simulink model "Mdl_Gear"  (R2024b)
settings: Solver=FixedStepDiscrete  StartTime=0.0  StopTime=10.0  FixedStep=0.1  RelTol=1e-3  EnableMultiTasking=on
values from neighbouring files (symbols this model uses):
  GEAR_MODE_OFF = mpt.Parameter    [Mdl_Gear_DD.m]
  GEAR_STATUS_OFF = mpt.Parameter    [Mdl_Gear_DD.m]
  HMI_READY = mpt.Parameter    [Mdl_Gear_DD.m]
  IND_FLASH_1HZ = mpt.Parameter    [Mdl_Gear_DD.m]
  IND_FLASH_4HZ = mpt.Parameter    [Mdl_Gear_DD.m]
  IND_TURN_OFF = mpt.Parameter    [Mdl_Gear_DD.m]
  Init_Count = mpt.Parameter    [Mdl_Gear_DD.m]
  Mdl_Gear_cTaskPeriod = mpt.Parameter    [Mdl_Gear_rte_types.m]
  PGM_LOGIC_ENABLE = mpt.Parameter    [Mdl_Gear_DD.m]
  RTE_E_MAX_AGE_EXCEEDED = mpt.Parameter    [Mdl_Gear_rte_types.m]
  RTE_E_NEVER_RECEIVED = mpt.Parameter    [Mdl_Gear_rte_types.m]
  Shift_Blink_P1 = mpt.Parameter    [Mdl_Gear_DD.m]
  Shift_Blink_P2 = mpt.Parameter    [Mdl_Gear_DD.m]
  STATUS_OFF = mpt.Parameter    [Mdl_Gear_DD.m]
  STATUS_ON = mpt.Parameter    [Mdl_Gear_DD.m]
  Timer_Param = mpt.Parameter    [Mdl_Gear_DD.m]
  TYPE1 = mpt.Parameter    [Mdl_Gear_DD.m]
  TYPE1_SBW = mpt.Parameter    [Mdl_Gear_DD.m]
  TYPE2 = mpt.Parameter    [Mdl_Gear_DD.m]
  TYPE2_MECH = mpt.Parameter    [Mdl_Gear_DD.m]
  TYPE3 = mpt.Parameter    [Mdl_Gear_DD.m]
  VALUE_FIFTEEN = mpt.Parameter    [Mdl_Gear_DD.m]
  VALUE_FIVE = mpt.Parameter    [Mdl_Gear_DD.m]
  VALUE_FOUR = mpt.Parameter    [Mdl_Gear_DD.m]
  VALUE_ONE = mpt.Parameter    [Mdl_Gear_DD.m]
  VALUE_TEN = mpt.Parameter    [Mdl_Gear_DD.m]
  VALUE_THREE = mpt.Parameter    [Mdl_Gear_DD.m]
  VALUE_TWO = mpt.Parameter    [Mdl_Gear_DD.m]
  VALUE_ZERO = mpt.Parameter    [Mdl_Gear_DD.m]
undefined symbols (not defined in the file or in its folder): CLUSTER_INACTIVE, eGearIn, eGearModeIn, eGearRecommendationIn, eGearStatusIn, eSIGNAL_MISSING, eSIGNAL_NEVER_RECEIVED, IgnOff, IgnOn, NETWORK_NORMAL, NETWORK_STANDALONE, PTSYS_EV, PTSYS_PHV, tRxSignalId_type_instance, tRxSignalStatus_type_instance
libraries: simulink x9
(part 1 of 2)
settings Model: Creator=AELANGO6  LastModifiedBy=AELANGO6
settings DataIOCC: SaveOutput=off
settings OptimizationCC: DefaultParameterBehavior=Inlined  EnhancedBackFolding=on  PassReuseOutputArgsAs=Individual arguments  ZeroExternalMemoryAtStartup=off  ZeroInternalMemoryAtStartup=off  MaxStackSize=750  RemoveLocalVariableInitialization=off  OptimizeBlockOrder=speed  DifferentSizesBufferReuse=on  OptimizationCustomize=off  EfficientTunableParamExpr=on
settings DebuggingCC: ParameterTunabilityLossMsg=error
settings SFSimCC: MATLABDynamicMemAlloc=off
settings RTWCC: Description=AUTOSAR  SystemTargetFile=autosar.tlc  GenCodeOnly=on  TemplateMakefile=ert_default_tmf  PortableWordSizes=on  DataTypeReplacement=CDataTypesFixedWidth
settings CodeAppCC: ForceParamTrailComments=on  IgnoreCustomStorageClasses=off  OperatorAnnotations=on  SimulinkDataObjDesc=on  SFDataObjDesc=on  InsertBlockDesc=on
settings STFCustomTargetCC: TargetLangStandard=C99 (ISO)  MultiwordLength=256  ParMdlRefBuildCompliant=on  CompOptLevelCompliant=on  IncludeMdlTerminateFcn=off  CombineOutputUpdateFcns=on  SuppressErrorStatus=on  ERTCustomFileBanners=on  SupportNonFinite=off  SupportComplex=off  SupportContinuousTime=off  SupportNonInlinedSFcns=off  RemoveResetFunc=on  ParenthesesLevel=Maximum  CastingMode=Standards  MATLABClassNameForMDSCustomization=Simulink.SoftwareTarget.ERTCustomization  AutosarCompliant=on  UseToolchainInfoCompliant=on  LookupTableObjectStructAxisOrder=2,1,3,4,...  LUTObjectStructOrderEvenSpacing=Size,Table,Breakpoints  SystemTargetFile=autosar.tlc
settings ERTTargetCC: TargetLangStandard=C99 (ISO)  ConcurrentExecutionCompliant=off  IncludeMdlTerminateFcn=off  SuppressErrorStatus=on  SupportNonFinite=off  SupportComplex=off  ParenthesesLevel=Maximum  CastingMode=Standards  ModelStepFunctionPrototypeControlCompliant=off  CPPClassGenCompliant=off  AutosarCompliant=on  LookupTableObjectStructAxisOrder=2,1,3,4,...  LUTObjectStructOrderEvenSpacing=Size,Table,Breakpoints  ERTCustomFileTemplate=example_file_process.tlc  ERTFilePackagingFormat=CompactWithDataFile  BooleanTrueId=TRUE  BooleanFalseId=FALSE

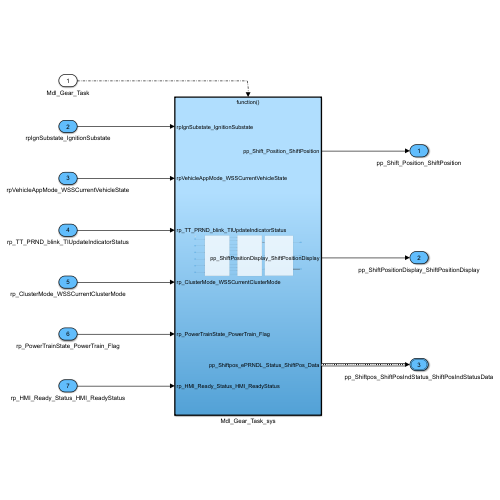
[thumbnail: Simulink's stored preview of the top-level diagram]
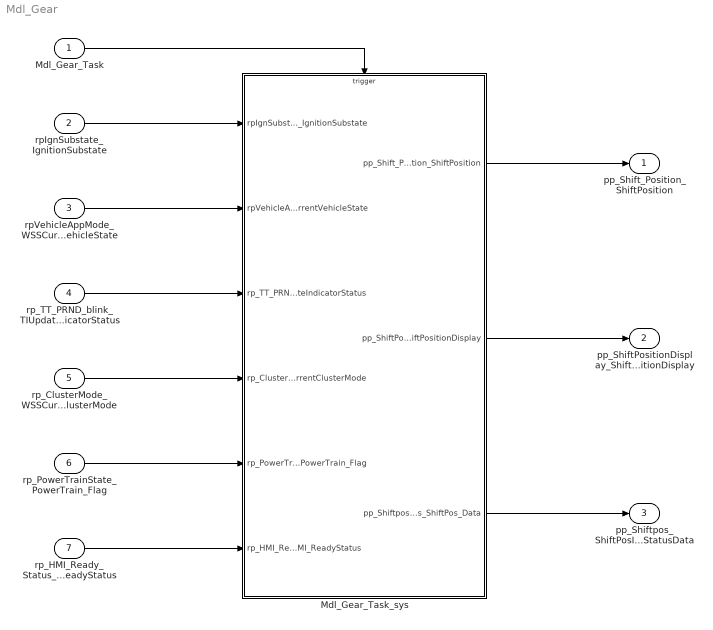
== system Mdl_Gear ==
  Mdl_Gear_Task : Inport  SampleTime=0.1  OutputFunctionCall=on
  rpIgnSubstate_IgnitionSubstate : Inport  Port=2  OutDataTypeStr=IgntionSubstateType  PortDimensions=1
  rpVehicleAppMode_WSSCurrentVehicleState : Inport  Port=3  OutDataTypeStr=VehicleActiveModes  PortDimensions=1
  rp_TT_PRND_blink_TIUpdateIndicatorStatus : Inport  Port=4  OutDataTypeStr=uint8  PortDimensions=1
  rp_ClusterMode_WSSCurrentClusterMode : Inport  Port=5  OutDataTypeStr=ClusterModes  PortDimensions=1
  rp_PowerTrainState_PowerTrain_Flag : Inport  Port=6  OutDataTypeStr=uint8  PortDimensions=1
  rp_HMI_Ready_Status_HMI_ReadyStatus : Inport  Port=7  OutDataTypeStr=HMIReadySts_Type  PortDimensions=1
  Mdl_Gear_Task_sys : Subsystem  TreatAsAtomicUnit=on
  pp_Shift_Position_ShiftPosition : Outport  OutDataTypeStr=ShiftPosition
  pp_ShiftPositionDisplay_ShiftPositionDisplay : Outport  Port=2  OutDataTypeStr=uint8
  pp_Shiftpos_ShiftPosIndStatus_ShiftPosIndStatusData : Outport  Port=3  OutDataTypeStr=Bus:SShiftPosIndStatus
  wires:
  Mdl_Gear_Task/1 -> Mdl_Gear_Task_sys/Trigger
  rp_ClusterMode_WSSCurrentClusterMode/1 -> Mdl_Gear_Task_sys/4(rp_ClusterMode_WSSCurrentClusterMode)
  rpIgnSubstate_IgnitionSubstate/1 -> Mdl_Gear_Task_sys/1(rpIgnSubstate_IgnitionSubstate)
  rpVehicleAppMode_WSSCurrentVehicleState/1 -> Mdl_Gear_Task_sys/2(rpVehicleAppMode_WSSCurrentVehicleState)
  Mdl_Gear_Task_sys/3(pp_Shiftpos_ePRNDL_Status_ShiftPos_Data) -> pp_Shiftpos_ShiftPosIndStatus_ShiftPosIndStatusData/1
  rp_TT_PRND_blink_TIUpdateIndicatorStatus/1 -> Mdl_Gear_Task_sys/3(rp_TT_PRND_blink_TIUpdateIndicatorStatus)
  Mdl_Gear_Task_sys/1(pp_Shift_Position_ShiftPosition) -> pp_Shift_Position_ShiftPosition/1
  rp_PowerTrainState_PowerTrain_Flag/1 -> Mdl_Gear_Task_sys/5(rp_PowerTrainState_PowerTrain_Flag)
  rp_HMI_Ready_Status_HMI_ReadyStatus/1 -> Mdl_Gear_Task_sys/6(rp_HMI_Ready_Status_HMI_ReadyStatus)
  Mdl_Gear_Task_sys/2(pp_ShiftPositionDisplay_ShiftPositionDisplay) -> pp_ShiftPositionDisplay_ShiftPositionDisplay/1

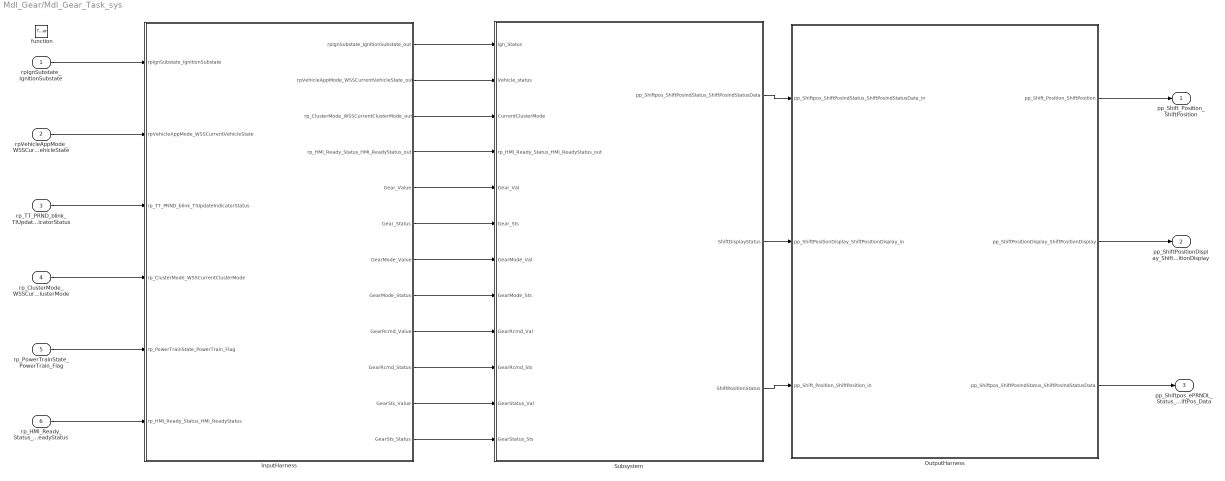
== system Mdl_Gear/Mdl_Gear_Task_sys ==
  rpIgnSubstate_IgnitionSubstate : Inport  OutDataTypeStr=IgntionSubstateType  PortDimensions=1
  rpVehicleAppMode_WSSCurrentVehicleState : Inport  Port=2  OutDataTypeStr=VehicleActiveModes  PortDimensions=1
  rp_TT_PRND_blink_TIUpdateIndicatorStatus : Inport  Port=3  OutDataTypeStr=uint8  PortDimensions=1
  rp_ClusterMode_WSSCurrentClusterMode : Inport  Port=4  OutDataTypeStr=ClusterModes  PortDimensions=1
  rp_PowerTrainState_PowerTrain_Flag : Inport  Port=5  OutDataTypeStr=uint8  PortDimensions=1
  rp_HMI_Ready_Status_HMI_ReadyStatus : Inport  Port=6  OutDataTypeStr=HMIReadySts_Type  PortDimensions=1
  function : TriggerPort  TriggerType=function-call  VariantControl=(inherit)  SampleTimeType=periodic  SampleTime=-1
  InputHarness : Subsystem  Variant=on
  OutputHarness : Subsystem  Variant=on
  Subsystem : Subsystem
  pp_Shift_Position_ShiftPosition : Outport  OutDataTypeStr=ShiftPosition  PortDimensions=1
  pp_ShiftPositionDisplay_ShiftPositionDisplay : Outport  Port=2  OutDataTypeStr=uint8  PortDimensions=1
  pp_Shiftpos_ePRNDL_Status_ShiftPos_Data : Outport  Port=3  OutDataTypeStr=Bus: SShiftPosIndStatus  PortDimensions=1
  wires:
  rpVehicleAppMode_WSSCurrentVehicleState/1 -> InputHarness/2(rpVehicleAppMode_WSSCurrentVehicleState)
  rpIgnSubstate_IgnitionSubstate/1 -> InputHarness/1(rpIgnSubstate_IgnitionSubstate)
  rp_TT_PRND_blink_TIUpdateIndicatorStatus/1 -> InputHarness/3(rp_TT_PRND_blink_TIUpdateIndicatorStatus)
  InputHarness/9(GearRcmd_Value) -> Subsystem/9(GearRcmd_Val)
  rp_ClusterMode_WSSCurrentClusterMode/1 -> InputHarness/4(rp_ClusterMode_WSSCurrentClusterMode)
  InputHarness/8(GearMode_Status) -> Subsystem/8(GearMode_Sts)
  rp_PowerTrainState_PowerTrain_Flag/1 -> InputHarness/5(rp_PowerTrainState_PowerTrain_Flag)
  rp_HMI_Ready_Status_HMI_ReadyStatus/1 -> InputHarness/6(rp_HMI_Ready_Status_HMI_ReadyStatus)
  InputHarness/1(rpIgnSubstate_IgnitionSubstate_out) -> Subsystem/1(Ign_Status)
  InputHarness/2(rpVehicleAppMode_WSSCurrentVehicleState_out) -> Subsystem/2(Vehicle_status)
  InputHarness/10(GearRcmd_Status) -> Subsystem/10(GearRcmd_Sts)
  InputHarness/3(rp_ClusterMode_WSSCurrentClusterMode_out) -> Subsystem/3(CurrentClusterMode)
  InputHarness/4(rp_HMI_Ready_Status_HMI_ReadyStatus_out) -> Subsystem/4(rp_HMI_Ready_Status_HMI_ReadyStatus_out)
  InputHarness/5(Gear_Value) -> Subsystem/5(Gear_Val)
  InputHarness/6(Gear_Status) -> Subsystem/6(Gear_Sts)
  InputHarness/7(GearMode_Value) -> Subsystem/7(GearMode_Val)
  InputHarness/11(GearSts_Value) -> Subsystem/11(GearStatus_Val)
  InputHarness/12(GearSts_Status) -> Subsystem/12(GearStatus_Sts)
  Subsystem/1(pp_Shiftpos_ShiftPosIndStatus_ShiftPosIndStatusData) -> OutputHarness/1(pp_Shiftpos_ShiftPosIndStatus_ShiftPosIndStatusData_in)
  Subsystem/2(ShiftDisplayStatus) -> OutputHarness/2(pp_ShiftPositionDisplay_ShiftPositionDisplay_in)
  Subsystem/3(ShiftPositionStatus) -> OutputHarness/3(pp_Shift_Position_ShiftPosition_in)
  OutputHarness/2(pp_ShiftPositionDisplay_ShiftPositionDisplay) -> pp_ShiftPositionDisplay_ShiftPositionDisplay/1
  OutputHarness/3(pp_Shiftpos_ShiftPosIndStatus_ShiftPosIndStatusData) -> pp_Shiftpos_ePRNDL_Status_ShiftPos_Data/1
  OutputHarness/1(pp_Shift_Position_ShiftPosition) -> pp_Shift_Position_ShiftPosition/1

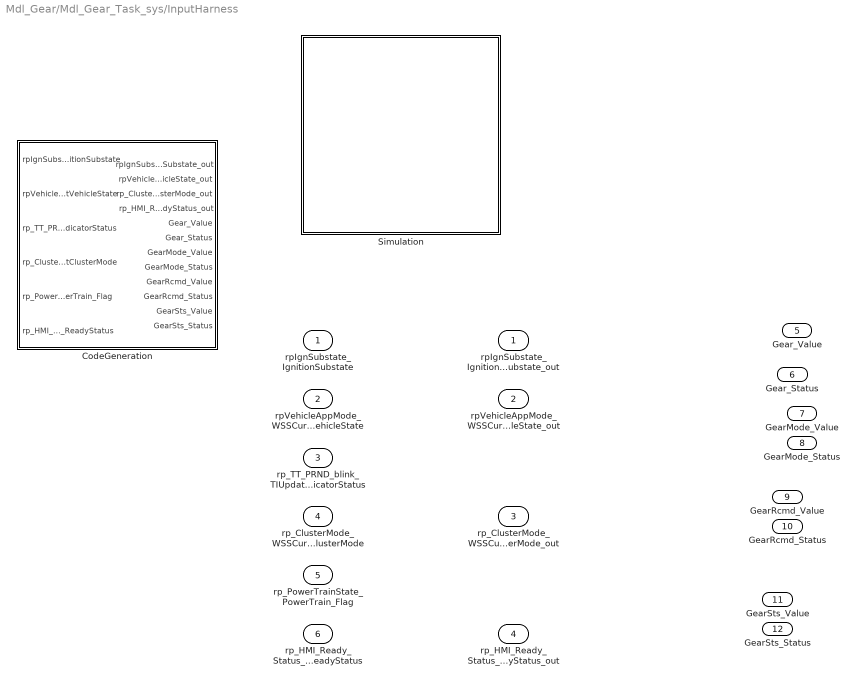
== system Mdl_Gear/Mdl_Gear_Task_sys/InputHarness ==
  rpIgnSubstate_IgnitionSubstate : Inport  OutDataTypeStr=IgntionSubstateType  PortDimensions=1
  rpVehicleAppMode_WSSCurrentVehicleState : Inport  Port=2  OutDataTypeStr=VehicleActiveModes  PortDimensions=1
  rp_TT_PRND_blink_TIUpdateIndicatorStatus : Inport  Port=3  OutDataTypeStr=uint8  PortDimensions=1
  rp_ClusterMode_WSSCurrentClusterMode : Inport  Port=4  OutDataTypeStr=ClusterModes  PortDimensions=1
  rp_PowerTrainState_PowerTrain_Flag : Inport  Port=5  OutDataTypeStr=uint8  PortDimensions=1
  rp_HMI_Ready_Status_HMI_ReadyStatus : Inport  Port=6  OutDataTypeStr=HMIReadySts_Type  PortDimensions=1
  CodeGeneration : Subsystem  VariantControl=CODEGENERATION
  Simulation : Subsystem  VariantControl=SIMULATION
  rpIgnSubstate_IgnitionSubstate_out : Outport  OutDataTypeStr=IgntionSubstateType  PortDimensions=1
  rpVehicleAppMode_WSSCurrentVehicleState_out : Outport  Port=2  OutDataTypeStr=VehicleActiveModes  PortDimensions=1
  rp_ClusterMode_WSSCurrentClusterMode_out : Outport  Port=3  OutDataTypeStr=ClusterModes  PortDimensions=1
  rp_HMI_Ready_Status_HMI_ReadyStatus_out : Outport  Port=4  OutDataTypeStr=HMIReadySts_Type  PortDimensions=1
  Gear_Value : Outport  Port=5
  Gear_Status : Outport  Port=6
  GearMode_Value : Outport  Port=7
  GearMode_Status : Outport  Port=8
  GearRcmd_Value : Outport  Port=9
  GearRcmd_Status : Outport  Port=10
  GearSts_Value : Outport  Port=11
  GearSts_Status : Outport  Port=12

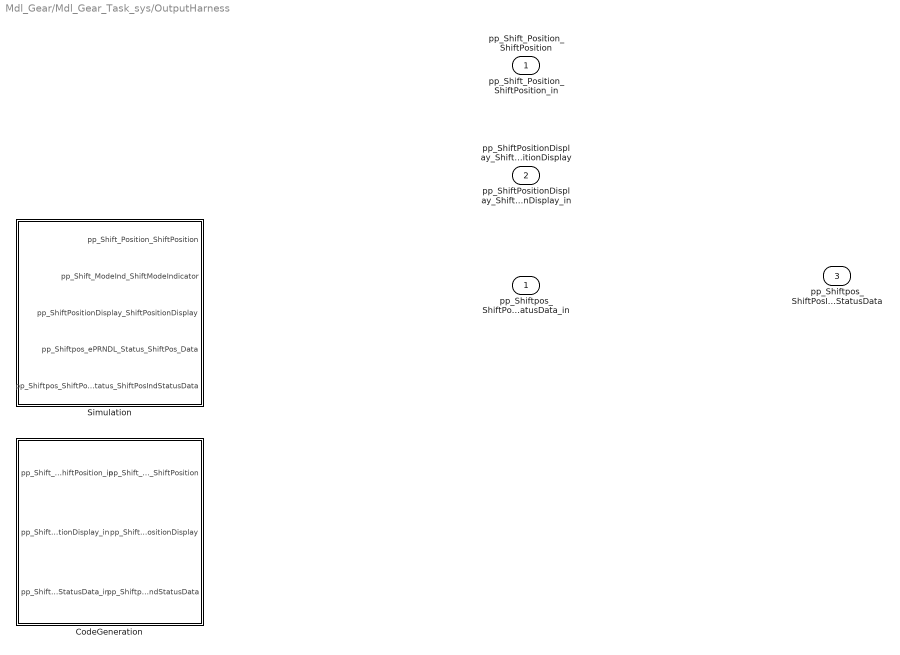
== system Mdl_Gear/Mdl_Gear_Task_sys/OutputHarness ==
  pp_Shiftpos_ShiftPosIndStatus_ShiftPosIndStatusData_in : Inport  OutDataTypeStr=Bus:SShiftPosIndStatus  PortDimensions=1
  pp_ShiftPositionDisplay_ShiftPositionDisplay_in : Inport  Port=2  OutDataTypeStr=uint8  PortDimensions=1
  pp_Shift_Position_ShiftPosition_in : Inport  Port=3  OutDataTypeStr=ShiftPosition  PortDimensions=1
  CodeGeneration : Subsystem  VariantControl=CODEGENERATION
  Simulation : Subsystem  VariantControl=SIMULATION
  pp_Shift_Position_ShiftPosition : Outport  OutDataTypeStr=ShiftPosition  PortDimensions=1
  pp_ShiftPositionDisplay_ShiftPositionDisplay : Outport  Port=2  OutDataTypeStr=uint8  PortDimensions=1
  pp_Shiftpos_ShiftPosIndStatus_ShiftPosIndStatusData : Outport  Port=3  OutDataTypeStr=Bus:SShiftPosIndStatus  PortDimensions=1

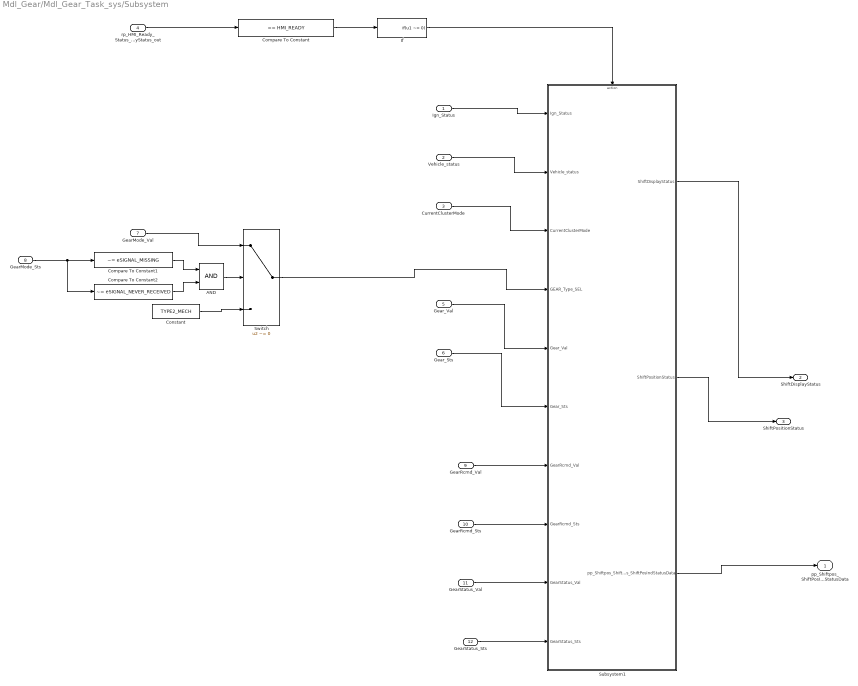
== system Mdl_Gear/Mdl_Gear_Task_sys/Subsystem ==
  Ign_Status : Inport
  Vehicle_status : Inport  Port=2
  CurrentClusterMode : Inport  Port=3
  rp_HMI_Ready_Status_HMI_ReadyStatus_out : Inport  Port=4
  Gear_Val : Inport  Port=5
  Gear_Sts : Inport  Port=6
  GearMode_Val : Inport  Port=7
  GearMode_Sts : Inport  Port=8
  GearRcmd_Val : Inport  Port=9
  GearRcmd_Sts : Inport  Port=10
  GearStatus_Val : Inport  Port=11
  GearStatus_Sts : Inport  Port=12
  AND : Logic  AllPortsSameDT=off  OutDataTypeStr=boolean
  Compare To Constant : simulink/Logic and Bit Operations/Compare To Constant  relop===  const=HMI_READY  OutDataTypeStr=boolean
  Compare To Constant1 : simulink/Logic and Bit Operations/Compare To Constant  relop=~=  const=eSIGNAL_MISSING  OutDataTypeStr=boolean
  Compare To Constant2 : simulink/Logic and Bit Operations/Compare To Constant  relop=~=  const=eSIGNAL_NEVER_RECEIVED  OutDataTypeStr=boolean
  Constant : Constant  Value=TYPE2_MECH
  If : If  IfExpression=u1 ~= 0  ShowElse=off
  Subsystem1 : Subsystem
  Switch : Switch  Criteria=u2 ~= 0  SaturateOnIntegerOverflow=off  InputSameDT=off
  pp_Shiftpos_ShiftPosIndStatus_ShiftPosIndStatusData : Outport  OutDataTypeStr=Bus:SShiftPosIndStatus  PortDimensions=1  VectorParamsAs1DForOutWhenUnconnected=off
  ShiftDisplayStatus : Outport  Port=2  VectorParamsAs1DForOutWhenUnconnected=off
  ShiftPositionStatus : Outport  Port=3  OutDataTypeStr=uint8  VectorParamsAs1DForOutWhenUnconnected=off
  wires:
  Ign_Status/1 -> Subsystem1/1(Ign_Status)
  CurrentClusterMode/1 -> Subsystem1/3(CurrentClusterMode)
  Subsystem1/3(pp_Shiftpos_ShiftPosIndStatus_ShiftPosIndStatusData) -> pp_Shiftpos_ShiftPosIndStatus_ShiftPosIndStatusData/1
  Subsystem1/1(ShiftDisplayStatus) -> ShiftDisplayStatus/1
  Subsystem1/2(ShiftPositionStatus) -> ShiftPositionStatus/1
  rp_HMI_Ready_Status_HMI_ReadyStatus_out/1 -> Compare To Constant/1
  Compare To Constant/1 -> If/1
  If/1 -> Subsystem1/Action
  Vehicle_status/1 -> Subsystem1/2(Vehicle_status)
  Gear_Val/1 -> Subsystem1/5(Gear_Val)
  Gear_Sts/1 -> Subsystem1/6(Gear_Sts)
  GearMode_Val/1 -> Switch/1
  GearMode_Sts/1 -> Compare To Constant2/1, Compare To Constant1/1
  GearRcmd_Val/1 -> Subsystem1/7(GearRcmd_Val)
  GearRcmd_Sts/1 -> Subsystem1/8(GearRcmd_Sts)
  GearStatus_Val/1 -> Subsystem1/9(GearStatus_Val)
  GearStatus_Sts/1 -> Subsystem1/10(GearStatus_Sts)
  Compare To Constant1/1 -> AND/1
  Compare To Constant2/1 -> AND/2
  AND/1 -> Switch/2
  Switch/1 -> Subsystem1/4(GEAR_Type_SEL)
  Constant/1 -> Switch/3

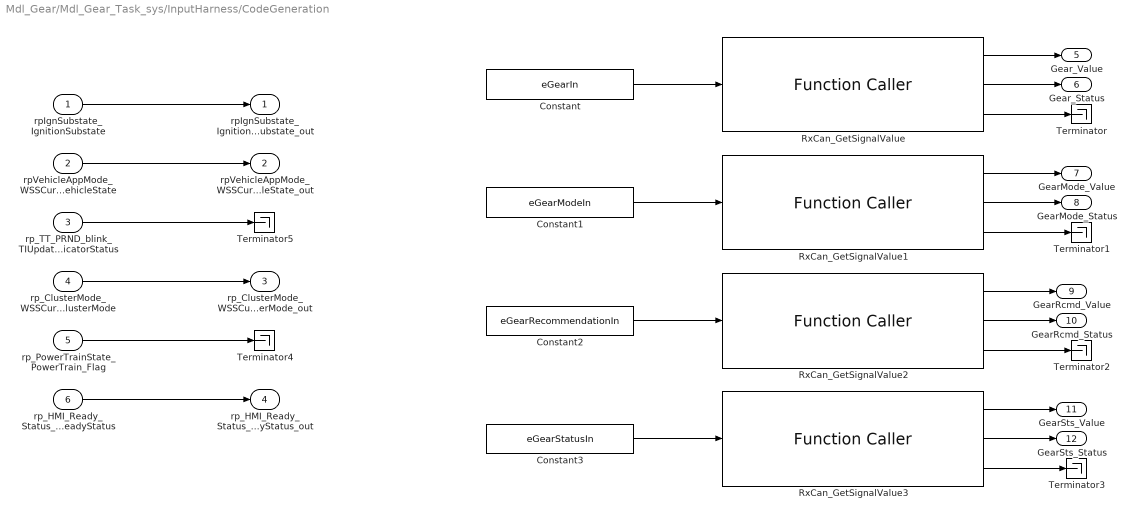
== system Mdl_Gear/Mdl_Gear_Task_sys/InputHarness/CodeGeneration ==
  rpIgnSubstate_IgnitionSubstate : Inport  OutDataTypeStr=IgntionSubstateType  PortDimensions=1
  rpVehicleAppMode_WSSCurrentVehicleState : Inport  Port=2  OutDataTypeStr=VehicleActiveModes  PortDimensions=1
  rp_TT_PRND_blink_TIUpdateIndicatorStatus : Inport  Port=3  OutDataTypeStr=uint8  PortDimensions=1
  rp_ClusterMode_WSSCurrentClusterMode : Inport  Port=4  OutDataTypeStr=ClusterModes  PortDimensions=1
  rp_PowerTrainState_PowerTrain_Flag : Inport  Port=5  OutDataTypeStr=uint8  PortDimensions=1
  rp_HMI_Ready_Status_HMI_ReadyStatus : Inport  Port=6  OutDataTypeStr=HMIReadySts_Type  PortDimensions=1
  Constant : Constant  Value=eGearIn
  Constant1 : Constant  Value=eGearModeIn
  Constant2 : Constant  Value=eGearRecommendationIn
  Constant3 : Constant  Value=eGearStatusIn
  RxCan_GetSignalValue{,1..3} (4 alike) : FunctionCaller  FunctionPrototype=[pSignalValue,pSignalStatus,error_status] = RxCan_GetSignalValue(SignalId)  InputArgumentSpecifications=tRxSignalId_type_instance(1)  OutputArgumentSpecifications=uint8(1) ,tRxSignalStatus_type_instance(1) ,uint8(1)
  Terminator{,1..5} (6 alike) : Terminator
  rpIgnSubstate_IgnitionSubstate_out : Outport  OutDataTypeStr=IgntionSubstateType  PortDimensions=1
  rpVehicleAppMode_WSSCurrentVehicleState_out : Outport  Port=2  OutDataTypeStr=VehicleActiveModes  PortDimensions=1
  rp_ClusterMode_WSSCurrentClusterMode_out : Outport  Port=3  OutDataTypeStr=ClusterModes  PortDimensions=1
  rp_HMI_Ready_Status_HMI_ReadyStatus_out : Outport  Port=4  OutDataTypeStr=HMIReadySts_Type  PortDimensions=1
  Gear_Value : Outport  Port=5
  Gear_Status : Outport  Port=6
  GearMode_Value : Outport  Port=7
  GearMode_Status : Outport  Port=8
  GearRcmd_Value : Outport  Port=9
  GearRcmd_Status : Outport  Port=10
  GearSts_Value : Outport  Port=11
  GearSts_Status : Outport  Port=12
  wires:
  rpIgnSubstate_IgnitionSubstate/1 -> rpIgnSubstate_IgnitionSubstate_out/1
  rpVehicleAppMode_WSSCurrentVehicleState/1 -> rpVehicleAppMode_WSSCurrentVehicleState_out/1
  rp_TT_PRND_blink_TIUpdateIndicatorStatus/1 -> Terminator5/1
  rp_ClusterMode_WSSCurrentClusterMode/1 -> rp_ClusterMode_WSSCurrentClusterMode_out/1
  rp_PowerTrainState_PowerTrain_Flag/1 -> Terminator4/1
  rp_HMI_Ready_Status_HMI_ReadyStatus/1 -> rp_HMI_Ready_Status_HMI_ReadyStatus_out/1
  Constant/1 -> RxCan_GetSignalValue/1
  Constant3/1 -> RxCan_GetSignalValue3/1
  Constant2/1 -> RxCan_GetSignalValue2/1
  Constant1/1 -> RxCan_GetSignalValue1/1
  RxCan_GetSignalValue/1 -> Gear_Value/1
  RxCan_GetSignalValue/2 -> Gear_Status/1
  RxCan_GetSignalValue/3 -> Terminator/1
  RxCan_GetSignalValue1/1 -> GearMode_Value/1
  RxCan_GetSignalValue1/3 -> Terminator1/1
  RxCan_GetSignalValue1/2 -> GearMode_Status/1
  RxCan_GetSignalValue2/1 -> GearRcmd_Value/1
  RxCan_GetSignalValue2/3 -> Terminator2/1
  RxCan_GetSignalValue2/2 -> GearRcmd_Status/1
  RxCan_GetSignalValue3/1 -> GearSts_Value/1
  RxCan_GetSignalValue3/3 -> Terminator3/1
  RxCan_GetSignalValue3/2 -> GearSts_Status/1

== system Mdl_Gear/Mdl_Gear_Task_sys/InputHarness/Simulation ==

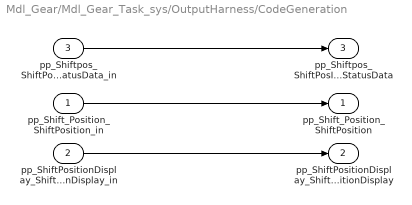
== system Mdl_Gear/Mdl_Gear_Task_sys/OutputHarness/CodeGeneration ==
  pp_Shift_Position_ShiftPosition_in : Inport  OutDataTypeStr=ShiftPosition  PortDimensions=1
  pp_ShiftPositionDisplay_ShiftPositionDisplay_in : Inport  Port=2  OutDataTypeStr=uint8  PortDimensions=1
  pp_Shiftpos_ShiftPosIndStatus_ShiftPosIndStatusData_in : Inport  Port=3  OutDataTypeStr=Bus:SShiftPosIndStatus  PortDimensions=1
  pp_Shift_Position_ShiftPosition : Outport  OutDataTypeStr=ShiftPosition  PortDimensions=1
  pp_ShiftPositionDisplay_ShiftPositionDisplay : Outport  Port=2  OutDataTypeStr=uint8  PortDimensions=1
  pp_Shiftpos_ShiftPosIndStatus_ShiftPosIndStatusData : Outport  Port=3  OutDataTypeStr=Bus:SShiftPosIndStatus  PortDimensions=1
  wires:
  pp_Shiftpos_ShiftPosIndStatus_ShiftPosIndStatusData_in/1 -> pp_Shiftpos_ShiftPosIndStatus_ShiftPosIndStatusData/1
  pp_ShiftPositionDisplay_ShiftPositionDisplay_in/1 -> pp_ShiftPositionDisplay_ShiftPositionDisplay/1
  pp_Shift_Position_ShiftPosition_in/1 -> pp_Shift_Position_ShiftPosition/1

== system Mdl_Gear/Mdl_Gear_Task_sys/OutputHarness/Simulation ==
  pp_Shift_Position_ShiftPosition : Outport  OutDataTypeStr=ShiftPosition  PortDimensions=1
  pp_Shift_ModeInd_ShiftModeIndicator : Outport  Port=2  OutDataTypeStr=ShiftPositionInd  PortDimensions=1
  pp_ShiftPositionDisplay_ShiftPositionDisplay : Outport  Port=3  OutDataTypeStr=uint8  PortDimensions=1
  pp_Shiftpos_ePRNDL_Status_ShiftPos_Data : Outport  Port=4  OutDataTypeStr=Bus:ShiftposData_Type  PortDimensions=1
  pp_Shiftpos_ShiftPosIndStatus_ShiftPosIndStatusData : Outport  Port=5  OutDataTypeStr=Bus:SShiftPosIndStatus  PortDimensions=1

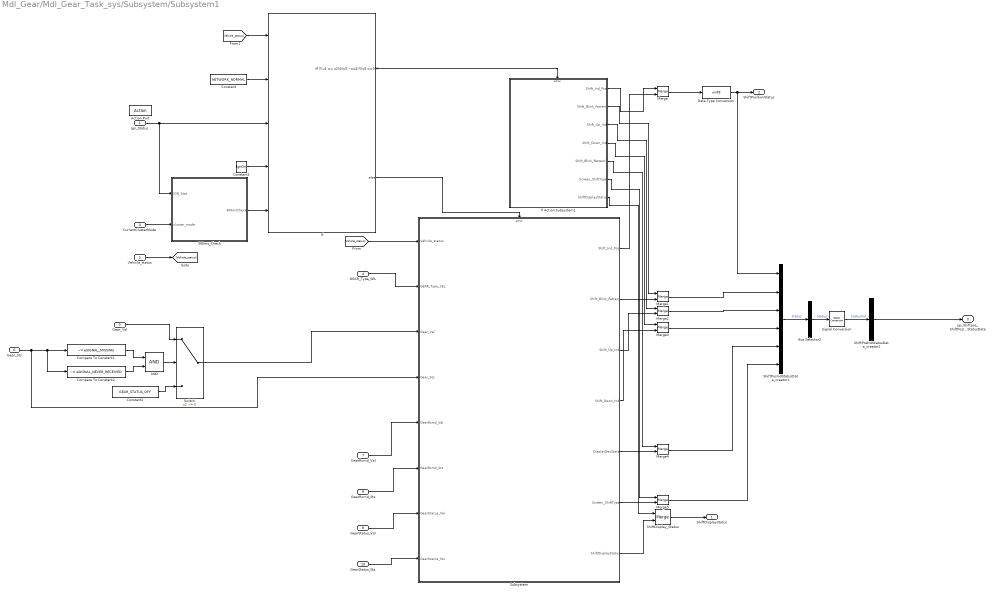
== system Mdl_Gear/Mdl_Gear_Task_sys/Subsystem/Subsystem1 ==
  Ign_Status : Inport
  Vehicle_status : Inport  Port=2
  CurrentClusterMode : Inport  Port=3
  GEAR_Type_SEL : Inport  Port=4
  Gear_Val : Inport  Port=5
  Gear_Sts : Inport  Port=6
  GearRcmd_Val : Inport  Port=7
  GearRcmd_Sts : Inport  Port=8
  GearStatus_Val : Inport  Port=9
  GearStatus_Sts : Inport  Port=10
  Action Port : ActionPort  ActionPortLabel=if(u1 ~= 0)
  300ms_Check : Subsystem
  AND : Logic  AllPortsSameDT=off  OutDataTypeStr=boolean
  Bus Selector2 : BusSelector  OutputSignals=Shift_Ind_Pos,Shift_Ind_BlinkReq,Shift_Ind_Up,Shift_Ind_Down,Shift_Ind_DisplayDecState,Shift_Ind_Screen_ShiftType  OutputAsBus=on
  Compare To Constant1 : simulink/Logic and Bit Operations/Compare To Constant  relop=~=  const=eSIGNAL_MISSING  OutDataTypeStr=boolean
  Compare To Constant2 : simulink/Logic and Bit Operations/Compare To Constant  relop=~=  const=eSIGNAL_NEVER_RECEIVED  OutDataTypeStr=boolean
  Constant : Constant  Value=NETWORK_NORMAL
  Constant1 : Constant  Value=IgnOn
  Constant2 : Constant  Value=GEAR_STATUS_OFF
  Data Type Conversion : DataTypeConversion  OutDataTypeStr=uint8  SaturateOnIntegerOverflow=off  RndMeth=Floor
  If : If  NumInputs=5  IfExpression=(((u1 == u2)&(u3 ~=u4))|(u5 ==0))
  If Action Subsystem1 : Subsystem  TreatAsAtomicUnit=on
  Merge{,1..5} (6 alike) : Merge
  ShiftDisplay_Status : Merge
  ShiftPosIndStatusData_creator1 : BusCreator  Inputs=6  OutDataTypeStr=Bus:SShiftInd  NonVirtualBus=on
      settings: InheritFromInputs=off
  ShiftPosIndStatusData_creator2 : BusCreator  Inputs=1  OutDataTypeStr=Bus:SShiftPosIndStatus  NonVirtualBus=on
      settings: InheritFromInputs=off
  Signal Conversion : SignalConversion  OverrideOpt=on
  Subsystem : Subsystem
  Switch : Switch  Criteria=u2 ~= 0  SaturateOnIntegerOverflow=off  InputSameDT=off
  ShiftDisplayStatus : Outport  VectorParamsAs1DForOutWhenUnconnected=off
  ShiftPositionStatus : Outport  Port=2  OutDataTypeStr=uint8  VectorParamsAs1DForOutWhenUnconnected=off
  pp_Shiftpos_ShiftPosIndStatus_ShiftPosIndStatusData : Outport  Port=3  OutDataTypeStr=Bus:SShiftPosIndStatus  PortDimensions=1  VectorParamsAs1DForOutWhenUnconnected=off
  wires:
  If/1 -> If Action Subsystem1/Action
  300ms_Check/1(300msCheck) -> If/5
  Constant1/1 -> If/4
  Ign_Status/1 -> If/3, 300ms_Check/1(IGN_Stat)
  [Vehicle_status] -> If/1
  CurrentClusterMode/1 -> 300ms_Check/2(cluster_mode)
  Vehicle_status/1 -> [Vehicle_status]
  Constant/1 -> If/2
  If/2 -> Subsystem/Action
  [Vehicle_status] -> Subsystem/1(Vehicle_status)
  GEAR_Type_SEL/1 -> Subsystem/2(GEAR_Type_SEL)
  GearRcmd_Val/1 -> Subsystem/5(GearRcmd_Val)
  If Action Subsystem1/7(ShiftDisplayStatus) -> ShiftDisplay_Status/1
  GearRcmd_Sts/1 -> Subsystem/6(GearRcmd_Sts)
  Subsystem/1(Shift_Ind_Pos) -> Merge/2
  GearStatus_Sts/1 -> Subsystem/8(GearStatus_Sts)
  GearStatus_Val/1 -> Subsystem/7(GearStatus_Val)
  If Action Subsystem1/1(Shift_Ind_Pos) -> Merge/1
  If Action Subsystem1/2(Shift_Blink_Pattern) -> Merge1/1
  If Action Subsystem1/3(Shift_Up_Ind) -> Merge2/1
  If Action Subsystem1/4(Shift_Down_Ind) -> Merge3/1
  If Action Subsystem1/5(Shift_Blink_Pattern3) -> Merge4/1
  If Action Subsystem1/6(Screen_ShiftType) -> Merge5/1
  Subsystem/2(Shift_Blink_Pattern) -> Merge1/2
  Subsystem/3(Shift_Up_Ind) -> Merge2/2
  Merge5/1 -> ShiftPosIndStatusData_creator1/6
  Subsystem/4(Shift_Down_Ind) -> Merge3/2
  Subsystem/5(DisplayDecState) -> Merge4/2
  Subsystem/6(Screen_ShiftType) -> Merge5/2
  Subsystem/7(ShiftDisplayStatus) -> ShiftDisplay_Status/2
  Merge/1 -> Data Type Conversion/1
  Merge1/1 -> ShiftPosIndStatusData_creator1/2
  Merge2/1 -> ShiftPosIndStatusData_creator1/3
  Merge3/1 -> ShiftPosIndStatusData_creator1/4
  Merge4/1 -> ShiftPosIndStatusData_creator1/5
  ShiftDisplay_Status/1 -> ShiftDisplayStatus/1
  Data Type Conversion/1 -> ShiftPosIndStatusData_creator1/1, ShiftPositionStatus/1
  Bus Selector2/1 -> Signal Conversion/1  "status"
  ShiftPosIndStatusData_creator2/1 -> pp_Shiftpos_ShiftPosIndStatus_ShiftPosIndStatusData/1
  Signal Conversion/1 -> ShiftPosIndStatusData_creator2/1  "statusInd"
  ShiftPosIndStatusData_creator1/1 -> Bus Selector2/1  "status"
  Constant2/1 -> Switch/3
  Compare To Constant2/1 -> AND/2
  Compare To Constant1/1 -> AND/1
  Gear_Val/1 -> Switch/1
  Switch/1 -> Subsystem/3(Gear_Val)
  AND/1 -> Switch/2
  Gear_Sts/1 -> Subsystem/4(Gear_Sts), Compare To Constant2/1, Compare To Constant1/1

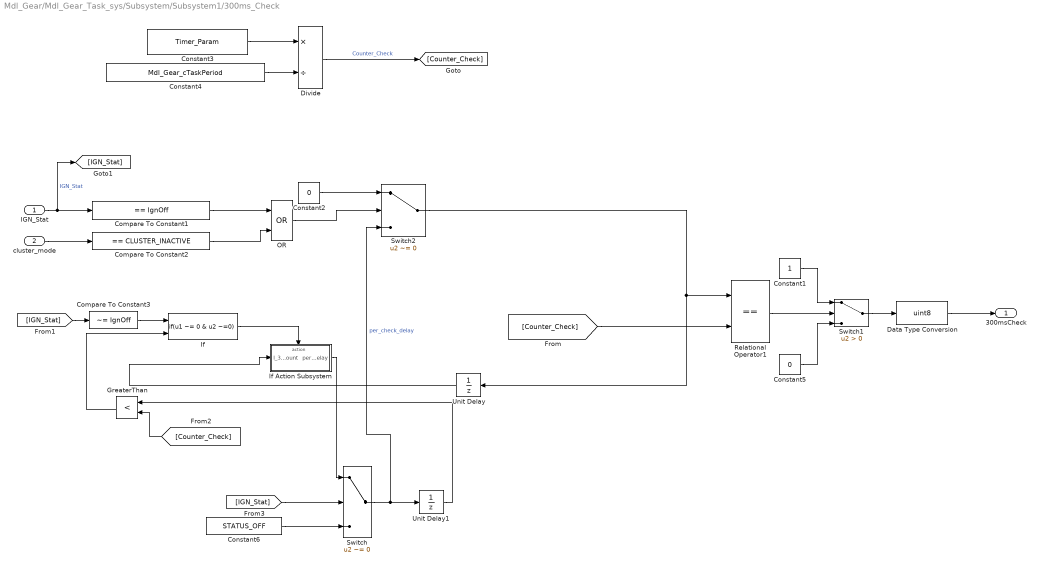
== system Mdl_Gear/Mdl_Gear_Task_sys/Subsystem/Subsystem1/300ms_Check ==
  IGN_Stat : Inport
  cluster_mode : Inport  Port=2
  Compare To Constant1 : simulink/Logic and Bit Operations/Compare To Constant  relop===  const=IgnOff  OutDataTypeStr=boolean
  Compare To Constant2 : simulink/Logic and Bit Operations/Compare To Constant  relop===  const=CLUSTER_INACTIVE  OutDataTypeStr=boolean
  Compare To Constant3 : simulink/Logic and Bit Operations/Compare To Constant  relop=~=  const=IgnOff  OutDataTypeStr=boolean
  Constant1 : Constant  OutDataTypeStr=uint8
  Constant2 : Constant  Value=0  OutDataTypeStr=uint8
  Constant3 : Constant  Value=Timer_Param  OutDataTypeStr=uint16
  Constant4 : Constant  Value=Mdl_Gear_cTaskPeriod
  Constant5 : Constant  Value=0  OutDataTypeStr=uint8
  Constant6 : Constant  Value=STATUS_OFF  OutDataTypeStr=uint16
  Data Type Conversion : DataTypeConversion  OutDataTypeStr=uint8  SaturateOnIntegerOverflow=off  RndMeth=Floor
  Divide : Product  Inputs=*/  OutDataTypeStr=fixdt('uint8', 'DataTypeOverride', 'Off')
  GreaterThan : RelationalOperator  Operator=<  OutDataTypeStr=boolean  RndMeth=Simplest  InputSameDT=off
  If : If  NumInputs=2  IfExpression=u1 ~= 0 & u2 ~=0  ShowElse=off
  If Action Subsystem : Subsystem  TreatAsAtomicUnit=on
  OR : Logic  Operator=OR  AllPortsSameDT=off  OutDataTypeStr=fixdt(0,8)
  Relational Operator1 : RelationalOperator  Operator===  OutDataTypeStr=boolean  RndMeth=Simplest  InputSameDT=off
  Switch : Switch  Criteria=u2 ~= 0  OutDataTypeStr=uint16  SaturateOnIntegerOverflow=off  InputSameDT=off
  Switch1 : Switch  Criteria=u2 > Threshold  SaturateOnIntegerOverflow=off  InputSameDT=off
  Switch2 : Switch  Criteria=u2 ~= 0  OutDataTypeStr=uint8  RndMeth=Simplest  SaturateOnIntegerOverflow=off  InputSameDT=off
  Unit Delay : UnitDelay  InitialCondition=Init_Count  SampleTime=-1  StateName=l_300ms_count  HasFrameUpgradeWarning=on
  Unit Delay1 : UnitDelay  SampleTime=-1  StateName=per_check_delay  HasFrameUpgradeWarning=on
  300msCheck : Outport  OutDataTypeStr=uint8  VectorParamsAs1DForOutWhenUnconnected=off
  wires:
  Constant2/1 -> Switch2/1
  Switch1/1 -> Data Type Conversion/1
  Constant1/1 -> Switch1/1
  Data Type Conversion/1 -> 300msCheck/1
  IGN_Stat/1 -> [IGN_Stat], Compare To Constant1/1  "IGN_Stat"
  [Counter_Check] -> Relational Operator1/2
  Constant5/1 -> Switch1/3
  Relational Operator1/1 -> Switch1/2
  Switch2/1 -> Unit Delay/1, Relational Operator1/1
  cluster_mode/1 -> Compare To Constant2/1
  OR/1 -> Switch2/2
  Compare To Constant2/1 -> OR/2
  Compare To Constant1/1 -> OR/1
  If/1 -> If Action Subsystem/Action
  Unit Delay/1 -> If Action Subsystem/1(l_300ms_count)
  [Counter_Check] -> GreaterThan/2
  GreaterThan/1 -> If/2
  Compare To Constant3/1 -> If/1
  Unit Delay1/1 -> GreaterThan/1
  Divide/1 -> [Counter_Check]  "Counter_Check"
  Constant4/1 -> Divide/2
  Constant3/1 -> Divide/1
  [IGN_Stat] -> Compare To Constant3/1
  Constant6/1 -> Switch/3
  [IGN_Stat] -> Switch/2
  If Action Subsystem/1(per_check_delay) -> Switch/1
  Switch/1 -> Switch2/3, Unit Delay1/1  "per_check_delay"

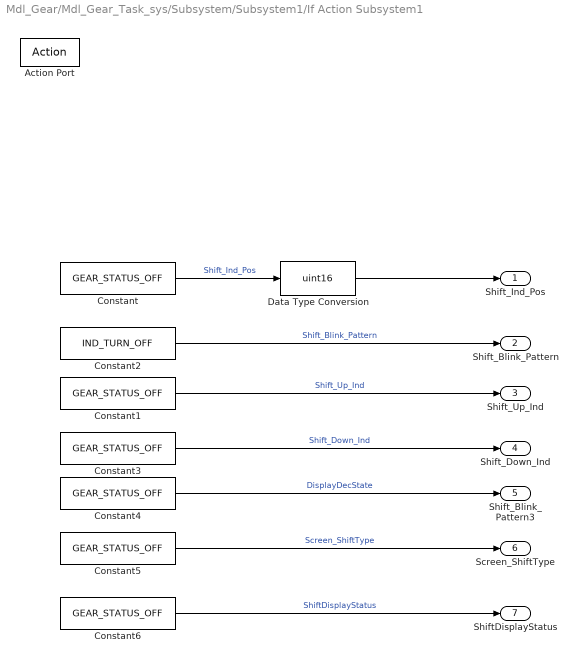
== system Mdl_Gear/Mdl_Gear_Task_sys/Subsystem/Subsystem1/If Action Subsystem1 ==
  Action Port : ActionPort  ActionPortLabel=if((((u1 == u2)&(u3 ~=u4))|(u5 ==0)))
  Constant : Constant  Value=GEAR_STATUS_OFF
  Constant{1,3..6} (5 alike) : Constant  Value=GEAR_STATUS_OFF  OutDataTypeStr=uint8
  Constant2 : Constant  Value=IND_TURN_OFF  OutDataTypeStr=uint8
  Data Type Conversion : DataTypeConversion  OutDataTypeStr=uint16  SaturateOnIntegerOverflow=off  RndMeth=Floor
  Shift_Ind_Pos : Outport  VectorParamsAs1DForOutWhenUnconnected=off
  Shift_Blink_Pattern : Outport  Port=2  VectorParamsAs1DForOutWhenUnconnected=off
  Shift_Up_Ind : Outport  Port=3  VectorParamsAs1DForOutWhenUnconnected=off
  Shift_Down_Ind : Outport  Port=4  VectorParamsAs1DForOutWhenUnconnected=off
  Shift_Blink_Pattern3 : Outport  Port=5  VectorParamsAs1DForOutWhenUnconnected=off
  Screen_ShiftType : Outport  Port=6  VectorParamsAs1DForOutWhenUnconnected=off
  ShiftDisplayStatus : Outport  Port=7  VectorParamsAs1DForOutWhenUnconnected=off
  wires:
  Constant5/1 -> Screen_ShiftType/1  "Screen_ShiftType"
  Constant2/1 -> Shift_Blink_Pattern/1  "Shift_Blink_Pattern"
  Constant6/1 -> ShiftDisplayStatus/1  "ShiftDisplayStatus"
  Constant1/1 -> Shift_Up_Ind/1  "Shift_Up_Ind"
  Constant3/1 -> Shift_Down_Ind/1  "Shift_Down_Ind"
  Constant4/1 -> Shift_Blink_Pattern3/1  "DisplayDecState"
  Constant/1 -> Data Type Conversion/1  "Shift_Ind_Pos"
  Data Type Conversion/1 -> Shift_Ind_Pos/1

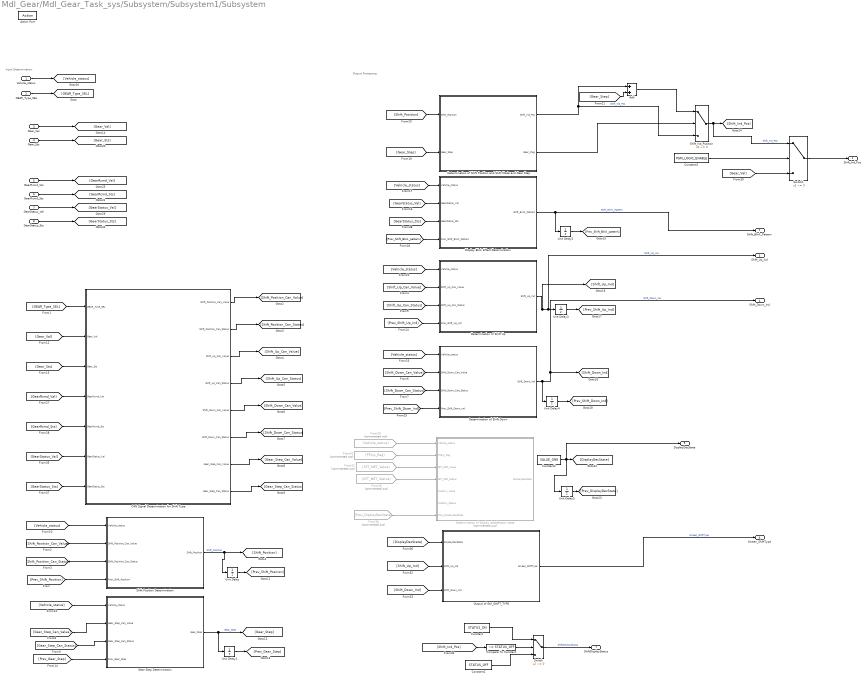
== system Mdl_Gear/Mdl_Gear_Task_sys/Subsystem/Subsystem1/Subsystem ==
  note: Input Determination
  note: Output Processing
  Vehicle_status : Inport
  GEAR_Type_SEL : Inport  Port=2
  Gear_Val : Inport  Port=3
  Gear_Sts : Inport  Port=4
  GearRcmd_Val : Inport  Port=5
  GearRcmd_Sts : Inport  Port=6
  GearStatus_Val : Inport  Port=7
  GearStatus_Sts : Inport  Port=8
  Action Port : ActionPort  ActionPortLabel=else
  Add : Sum  OutDataTypeStr=uint8  AccumDataTypeStr=fixdt('uint8', 'DataTypeOverride', 'Off')  RndMeth=Simplest  LockScale=on
  CAN Signal Determination for Shift Type : Subsystem
  Compare To Constant : simulink/Logic and Bit Operations/Compare To Constant  relop=~=  const=STATUS_OFF  OutDataTypeStr=boolean
  Constant : Constant  Value=STATUS_ON  OutDataTypeStr=uint8
  Constant1 : Constant  Value=STATUS_OFF  OutDataTypeStr=uint8
  Constant2 : Constant  Value=VALUE_ONE
  Constant3 : Constant  Value=PGM_LOGIC_ENABLE
  Determination of Display deceleration state : Truth Table  Commented=on  TreatAsAtomicUnit=on
  Determination of Shift Down : Truth Table  TreatAsAtomicUnit=on
  Determination of Shift Position and Shift Mode and Gear Step : Truth Table  TreatAsAtomicUnit=on
  Determination of Shift Up : Truth Table  TreatAsAtomicUnit=on
  Display Blink Effect Determination : Truth Table  TreatAsAtomicUnit=on
  From22 : From  Commented=on  GotoTag=SFT_MET_Value
  From26 : From  Commented=on  GotoTag=SFT_MET_Status
  From29 : From  Commented=on  GotoTag=Vehicle_status
  From30 : From  Commented=on  GotoTag=Prev_DisplayDecState
  From31 : From  Commented=on  GotoTag=PTSys_flag
  Gear Step Determination : Truth Table  TreatAsAtomicUnit=on
  Output of GUI_SHIFT_TYPE : Truth Table  TreatAsAtomicUnit=on
  Shift Position Determination : Truth Table  TreatAsAtomicUnit=on
  Shift_Ind_Position : Switch  Criteria=u2 ~= 0  Threshold=STATUS_OFF  OutDataTypeStr=uint16  SaturateOnIntegerOverflow=off  InputSameDT=off
  Switch : Switch  Criteria=u2 ~= 0  SaturateOnIntegerOverflow=off  InputSameDT=off
  Switch1 : Switch  Criteria=u2 ~= 0  SaturateOnIntegerOverflow=off  InputSameDT=off
  Unit Delay : UnitDelay  SampleTime=-1  StateName=Prev_Shift_Position  HasFrameUpgradeWarning=on
  Unit Delay1 : UnitDelay  SampleTime=-1  StateName=Prev_Gear_Step  HasFrameUpgradeWarning=on
  Unit Delay2 : UnitDelay  SampleTime=-1  StateName=Prev_Shift_Blink_pattern  HasFrameUpgradeWarning=on
  Unit Delay3 : UnitDelay  SampleTime=-1  StateName=Prev_Shift_Up_Ind  HasFrameUpgradeWarning=on
  Unit Delay4 : UnitDelay  SampleTime=-1  StateName=Prev_Shift_Down_Ind  HasFrameUpgradeWarning=on
  Unit Delay5 : UnitDelay  SampleTime=-1  StateName=Prev_DisplayDecState  HasFrameUpgradeWarning=on
  Shift_Ind_Pos : Outport  VectorParamsAs1DForOutWhenUnconnected=off
  Shift_Blink_Pattern : Outport  Port=2  VectorParamsAs1DForOutWhenUnconnected=off
  Shift_Up_Ind : Outport  Port=3  VectorParamsAs1DForOutWhenUnconnected=off
  Shift_Down_Ind : Outport  Port=4  VectorParamsAs1DForOutWhenUnconnected=off
  DisplayDecState : Outport  Port=5  VectorParamsAs1DForOutWhenUnconnected=off
  Screen_ShiftType : Outport  Port=6  VectorParamsAs1DForOutWhenUnconnected=off
  ShiftDisplayStatus : Outport  Port=7  OutDataTypeStr=uint8  VectorParamsAs1DForOutWhenUnconnected=off
  wires:
  GEAR_Type_SEL/1 -> [GEAR_Type_SEL]
  [GEAR_Type_SEL] -> CAN Signal Determination for Shift Type/1(GEAR_Type_SEL)
  CAN Signal Determination for Shift Type/1(" Shift_Position_Can_Value") -> [Shift_Position_Can_Value]
  CAN Signal Determination for Shift Type/2(Shift_Position_Can_Status) -> [Shift_Position_Can_Status]
  CAN Signal Determination for Shift Type/3(Shift_Up_Can_Value) -> [Shift_Up_Can_Value]
  CAN Signal Determination for Shift Type/4(Shift_Up_Can_Status) -> [Shift_Up_Can_Status]
  CAN Signal Determination for Shift Type/5(Shift_Down_Can_Value) -> [Shift_Down_Can_Value]
  CAN Signal Determination for Shift Type/6(Shift_Down_Can_Status) -> [Shift_Down_Can_Status]
  CAN Signal Determination for Shift Type/7(Gear_Step_Can_Value) -> [Gear_Step_Can_Value]
  CAN Signal Determination for Shift Type/8(Gear_Step_Can_Status) -> [Gear_Step_Can_Status]
  Vehicle_status/1 -> [Vehicle_status]
  [Shift_Position_Can_Status] -> Shift Position Determination/3(Shift_Position_Can_Status)
  Shift Position Determination/1(Shift_Position) -> Unit Delay/1, [Shift_Position]  "Shift_Position"
  [Shift_Position_Can_Value] -> Shift Position Determination/2(Shift_Position_Can_Value)
  [Vehicle_status] -> Shift Position Determination/1(Vehicle_status)
  Unit Delay/1 -> [Prev_Shift_Position]
  [Prev_Shift_Position] -> Shift Position Determination/4(Prev_Shift_Position)
  Unit Delay1/1 -> [Prev_Gear_Step]
  Gear Step Determination/1(Gear_Step) -> Unit Delay1/1, [Gear_Step]  "Gear_Step"
  [Gear_Step_Can_Status] -> Gear Step Determination/3(Gear_Step_Can_Status)
  [Gear_Step_Can_Value] -> Gear Step Determination/2(Gear_Step_Can_Value)
  [Vehicle_status] -> Gear Step Determination/1(Vehicle_status)
  [Prev_Gear_Step] -> Gear Step Determination/4(Prev_Gear_Step)
  [Vehicle_status] -> Display Blink Effect Determination/1(Vehicle_status)
  Display Blink Effect Determination/1(Shift_Blink_Pattern) -> Shift_Blink_Pattern/1, Unit Delay2/1  "Shift_Blink_Pattern"
  Unit Delay2/1 -> [Prev_Shift_Blink_pattern]
  [Prev_Shift_Blink_pattern] -> Display Blink Effect Determination/4(Prev_Shift_Blink_Pattern)
  [Gear_Step] -> Determination of Shift Position and Shift Mode and Gear Step/2(Gear_Step)
  [Shift_Position] -> Determination of Shift Position and Shift Mode and Gear Step/1(Shift_Position)
  Determination of Shift Up/1(Shift_Up_Ind) -> [Shift_Up_Ind], Shift_Up_Ind/1, Unit Delay3/1  "Shift_Up_Ind"
  Unit Delay3/1 -> [Prev_Shift_Up_Ind]
  [Shift_Up_Can_Value] -> Determination of Shift Up/2(Shift_Up_Can_Value)
  [Shift_Up_Can_Status] -> Determination of Shift Up/3(Shift_Up_Can_Status)
  [Vehicle_status] -> Determination of Shift Up/1(Vehicle_status)
  [Prev_Shift_Up_Ind] -> Determination of Shift Up/4(Prev_Shift_Up_Ind)
  Unit Delay4/1 -> [Prev_Shift_Down_Ind]
  [Prev_Shift_Down_Ind] -> Determination of Shift Down/4(Prev_Shift_Down_Ind)
  Determination of Shift Down/1(Shift_Down_Ind) -> Shift_Down_Ind/1, [Shift_Down_Ind], Unit Delay4/1  "Shift_Down_Ind"
  [Vehicle_status] -> Determination of Shift Down/1(Vehicle_status)
  [Shift_Down_Can_Status] -> Determination of Shift Down/3(Shift_Down_Can_Status)
  [Shift_Down_Can_Value] -> Determination of Shift Down/2(Shift_Down_Can_Value)
  From29/1 -> Determination of Display deceleration state/1(Vehicle_status)
  From22/1 -> Determination of Display deceleration state/3(SFT_MET_Value)
  From31/1 -> Determination of Display deceleration state/2(PTSys_flag)
  Unit Delay5/1 -> [Prev_DisplayDecState]
  From30/1 -> Determination of Display deceleration state/7(Prev_DisplayDecState)
  [Shift_Up_Ind] -> Output of GUI_SHIFT_TYPE/2(Shift_Up_Ind)
  Output of GUI_SHIFT_TYPE/1(Screen_ShiftType) -> Screen_ShiftType/1  "Screen_ShiftType"
  [DisplayDecState] -> Output of GUI_SHIFT_TYPE/1(DisplayDecState)
  [Shift_Down_Ind] -> Output of GUI_SHIFT_TYPE/3(Shift_Down_Ind)
  [Shift_Ind_Pos] -> Compare To Constant/1
  Compare To Constant/1 -> Switch/2
  Constant/1 -> Switch/1
  Constant1/1 -> Switch/3
  Switch/1 -> ShiftDisplayStatus/1  "ShiftDisplayStatus"
  From26/1 -> Determination of Display deceleration state/4(SFT_MET_Status)
  Determination of Shift Position and Shift Mode and Gear Step/1(Shift_Ind_Pos) -> Add/1, Shift_Ind_Position/3  "Shift_Ind_Pos"
  Shift_Ind_Position/1 -> Switch1/1, [Shift_Ind_Pos]  "Shift_Ind_Pos"
  Determination of Shift Position and Shift Mode and Gear Step/2(Gear_Flag) -> Shift_Ind_Position/2
  Add/1 -> Shift_Ind_Position/1
  [Gear_Step] -> Add/2
  Gear_Val/1 -> [Gear_Val]
  Gear_Sts/1 -> [Gear_Sts]
  GearRcmd_Val/1 -> [GearRcmd_Val]
  GearRcmd_Sts/1 -> [GearRcmd_Sts]
  GearStatus_Val/1 -> [GearStatus_Val]
  GearStatus_Sts/1 -> [GearStatus_Sts]
  [GearStatus_Val] -> CAN Signal Determination for Shift Type/6(GearStatus_Val)
  [GearRcmd_Val] -> CAN Signal Determination for Shift Type/4(GearRcmd_Val)
  [Gear_Sts] -> CAN Signal Determination for Shift Type/3(Gear_Sts)
  [GearStatus_Sts] -> CAN Signal Determination for Shift Type/7(GearStatus_Sts)
  [GearRcmd_Sts] -> CAN Signal Determination for Shift Type/5(GearRcmd_Sts)
  [Gear_Val] -> CAN Signal Determination for Shift Type/2(Gear_Val)
  [GearStatus_Val] -> Display Blink Effect Determination/2(GearStatus_Val)
  [GearStatus_Sts] -> Display Blink Effect Determination/3(GearStatus_Sts)
  Constant2/1 -> DisplayDecState/1, Unit Delay5/1, [DisplayDecState]
  Switch1/1 -> Shift_Ind_Pos/1
  [Gear_Val] -> Switch1/3
  Constant3/1 -> Switch1/2

== system Mdl_Gear/Mdl_Gear_Task_sys/Subsystem/Subsystem1/300ms_Check/If Action Subsystem ==
  l_300ms_count : Inport
  Action Port : ActionPort  ActionPortLabel=if(u1 ~= 0 & u2 ~=0)
  Add : Sum  OutDataTypeStr=uint16  AccumDataTypeStr=uint16
  Constant : Constant  Value=STATUS_ON  OutDataTypeStr=uint8
  per_check_delay : Outport  OutDataTypeStr=uint16  VectorParamsAs1DForOutWhenUnconnected=off
  wires:
  l_300ms_count/1 -> Add/2
  Constant/1 -> Add/1
  Add/1 -> per_check_delay/1

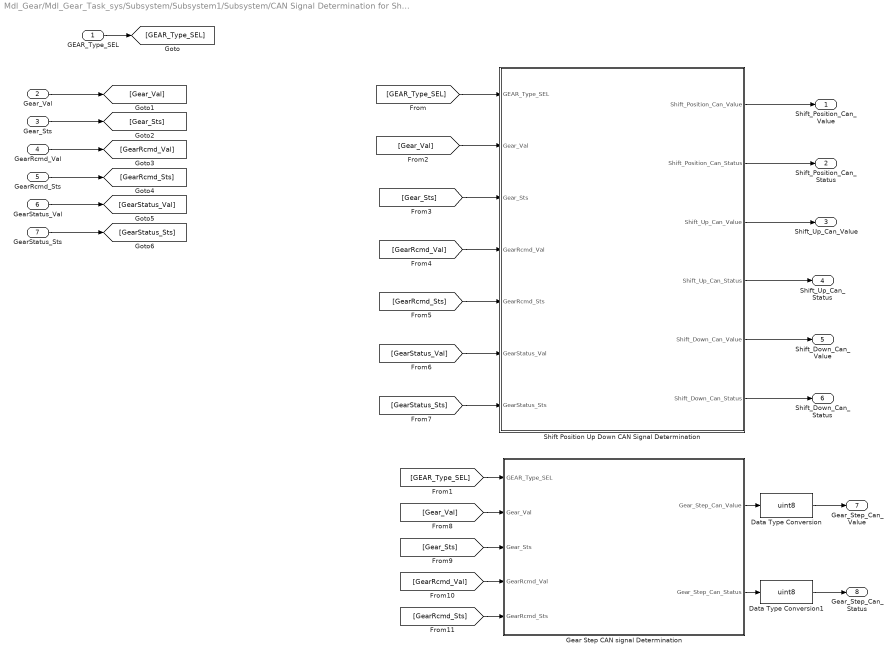
== system Mdl_Gear/Mdl_Gear_Task_sys/Subsystem/Subsystem1/Subsystem/CAN Signal Determination for Shift Type ==
  GEAR_Type_SEL : Inport
  Gear_Val : Inport  Port=2
  Gear_Sts : Inport  Port=3
  GearRcmd_Val : Inport  Port=4
  GearRcmd_Sts : Inport  Port=5
  GearStatus_Val : Inport  Port=6
  GearStatus_Sts : Inport  Port=7
  Data Type Conversion : DataTypeConversion  OutDataTypeStr=uint8  SaturateOnIntegerOverflow=off  RndMeth=Floor
  Data Type Conversion1 : DataTypeConversion  OutDataTypeStr=uint8  SaturateOnIntegerOverflow=off  RndMeth=Floor
  Gear Step CAN signal Determination : Truth Table  TreatAsAtomicUnit=on
  Shift Position Up Down CAN Signal Determination : Truth Table  TreatAsAtomicUnit=on
  " Shift_Position_Can_Value" : Outport  VectorParamsAs1DForOutWhenUnconnected=off
  Shift_Position_Can_Status : Outport  Port=2  VectorParamsAs1DForOutWhenUnconnected=off
  Shift_Up_Can_Value : Outport  Port=3  VectorParamsAs1DForOutWhenUnconnected=off
  Shift_Up_Can_Status : Outport  Port=4  VectorParamsAs1DForOutWhenUnconnected=off
  Shift_Down_Can_Value : Outport  Port=5  VectorParamsAs1DForOutWhenUnconnected=off
  Shift_Down_Can_Status : Outport  Port=6  VectorParamsAs1DForOutWhenUnconnected=off
  Gear_Step_Can_Value : Outport  Port=7  VectorParamsAs1DForOutWhenUnconnected=off
  Gear_Step_Can_Status : Outport  Port=8  VectorParamsAs1DForOutWhenUnconnected=off
  wires:
  Gear Step CAN signal Determination/1(Gear_Step_Can_Value) -> Data Type Conversion/1
  GEAR_Type_SEL/1 -> [GEAR_Type_SEL]
  [GEAR_Type_SEL] -> Shift Position Up Down CAN Signal Determination/1(GEAR_Type_SEL)
  [GEAR_Type_SEL] -> Gear Step CAN signal Determination/1(GEAR_Type_SEL)
  Data Type Conversion/1 -> Gear_Step_Can_Value/1
  Gear Step CAN signal Determination/2(Gear_Step_Can_Status) -> Data Type Conversion1/1
  Data Type Conversion1/1 -> Gear_Step_Can_Status/1
  Shift Position Up Down CAN Signal Determination/1(Shift_Position_Can_Value) -> " Shift_Position_Can_Value"/1
  Shift Position Up Down CAN Signal Determination/2(Shift_Position_Can_Status) -> Shift_Position_Can_Status/1
  Shift Position Up Down CAN Signal Determination/3(Shift_Up_Can_Value) -> Shift_Up_Can_Value/1
  Shift Position Up Down CAN Signal Determination/6(Shift_Down_Can_Status) -> Shift_Down_Can_Status/1
  Shift Position Up Down CAN Signal Determination/5(Shift_Down_Can_Value) -> Shift_Down_Can_Value/1
  Shift Position Up Down CAN Signal Determination/4(Shift_Up_Can_Status) -> Shift_Up_Can_Status/1
  Gear_Val/1 -> [Gear_Val]
  GearRcmd_Val/1 -> [GearRcmd_Val]
  GearRcmd_Sts/1 -> [GearRcmd_Sts]
  Gear_Sts/1 -> [Gear_Sts]
  GearStatus_Sts/1 -> [GearStatus_Sts]
  GearStatus_Val/1 -> [GearStatus_Val]
  [Gear_Val] -> Shift Position Up Down CAN Signal Determination/2(Gear_Val)
  [Gear_Sts] -> Shift Position Up Down CAN Signal Determination/3(Gear_Sts)
  [GearStatus_Sts] -> Shift Position Up Down CAN Signal Determination/7(GearStatus_Sts)
  [GearStatus_Val] -> Shift Position Up Down CAN Signal Determination/6(GearStatus_Val)
  [GearRcmd_Sts] -> Shift Position Up Down CAN Signal Determination/5(GearRcmd_Sts)
  [GearRcmd_Val] -> Shift Position Up Down CAN Signal Determination/4(GearRcmd_Val)
  [Gear_Val] -> Gear Step CAN signal Determination/2(Gear_Val)
  [Gear_Sts] -> Gear Step CAN signal Determination/3(Gear_Sts)
  [GearRcmd_Val] -> Gear Step CAN signal Determination/4(GearRcmd_Val)
  [GearRcmd_Sts] -> Gear Step CAN signal Determination/5(GearRcmd_Sts)

== matlab function Mdl_Gear/Mdl_Gear_Task_sys/Subsystem/Subsystem1/Subsystem/CAN Signal Determination for Shift Type/Gear Step CAN signal Determination ==
  data: GEAR_Type_SEL input uint8; Gear_Step_Can_Value output uint8; GEAR_STATUS_OFF parameter; Gear_Val input uint8; Gear_Sts input uint8; Gear_Step_Can_Status output uint8; GearRcmd_Val input uint8; GearRcmd_Sts input uint8; TYPE1_SBW parameter; TYPE2_MECH parameter; VALUE_ZERO parameter; eSIGNAL_MISSING parameter; VALUE_ONE parameter; VALUE_TEN parameter
function [Gear_Step_Can_Value, Gear_Step_Can_Status] = fcn(GEAR_Type_SEL, GEAR_STATUS_OFF, Gear_Val, Gear_Sts, GearRcmd_Val, GearRcmd_Sts, TYPE1_SBW, TYPE2_MECH, VALUE_ZERO, eSIGNAL_MISSING, VALUE_ONE, VALUE_TEN)

aVarTruthTableCondition_1 = false;
aVarTruthTableCondition_2 = false;


% Check Shift type 1

aVarTruthTableCondition_1 = logical(GEAR_Type_SEL ==TYPE1_SBW);

% Check Shift type 2

aVarTruthTableCondition_2 = logical(((GEAR_Type_SEL == TYPE2_MECH) && ((Gear_Val>= VALUE_ONE) && (Gear_Val<= VALUE_TEN))));

if (aVarTruthTableCondition_1)
    aFcnTruthTableAction_1();
elseif (aVarTruthTableCondition_2)
    aFcnTruthTableAction_2();
else % Default
    aFcnTruthTableAction_3();
end

function aFcnTruthTableAction_1()

% Type 1 : SBW

Gear_Step_Can_Value = Gear_Val;
Gear_Step_Can_Status = Gear_Sts;

function aFcnTruthTableAction_2()

% Type 2 : Mechanical shift

Gear_Step_Can_Value = Gear_Val;
Gear_Step_Can_Status = Gear_Sts;

function aFcnTruthTableAction_3()

% Others

Gear_Step_Can_Value = VALUE_ZERO;
Gear_Step_Can_Status = eSIGNAL_MISSING;

== matlab function Mdl_Gear/Mdl_Gear_Task_sys/Subsystem/Subsystem1/Subsystem/Shift Position Determination ==
  data: Vehicle_status input; Shift_Position output uint8; STATUS_OFF parameter; Shift_Position_Can_Value input; Shift_Position_Can_Status input; NETWORK_NORMAL parameter; NETWORK_STANDALONE parameter; eSIGNAL_NEVER_RECEIVED parameter; eSIGNAL_MISSING parameter; Prev_Shift_Position input uint8; Shift_Pos_RANGE_P parameter; Shift_Pos_RANGE_R parameter; Shift_Pos_RANGE_N parameter; Shift_Pos_RANGE_D parameter; Shift_Pos_RANGE_B parameter; Shift_Pos_RANGE_M parameter; Shift_Pos_RANGE_S parameter; Shift_Pos_RANGE_SD parameter; VALUE_ONE parameter; VALUE_TWO parameter; VALUE_THREE parameter; VALUE_FOUR parameter; VALUE_FIVE parameter; VALUE_SIX parameter; VALUE_SEVEN parameter; VALUE_EIGHT parameter
function Shift_Position = fcn(Vehicle_status, STATUS_OFF, Shift_Position_Can_Value, Shift_Position_Can_Status, NETWORK_NORMAL, NETWORK_STANDALONE, eSIGNAL_NEVER_RECEIVED, eSIGNAL_MISSING, Prev_Shift_Position, Shift_Pos_RANGE_P, Shift_Pos_RANGE_R, Shift_Pos_RANGE_N, Shift_Pos_RANGE_D, Shift_Pos_RANGE_B, Shift_Pos_RANGE_M, Shift_Pos_RANGE_S, Shift_Pos_RANGE_SD, VALUE_ONE, VALUE_TWO, VALUE_THREE, VALUE_FOUR, VALUE_FIVE, VALUE_SIX, VALUE_SEVEN, VALUE_EIGHT)

aVarTruthTableCondition_1 = false;
aVarTruthTableCondition_2 = false;
aVarTruthTableCondition_3 = false;
aVarTruthTableCondition_4 = false;
aVarTruthTableCondition_5 = false;
aVarTruthTableCondition_6 = false;
aVarTruthTableCondition_7 = false;
aVarTruthTableCondition_8 = false;
aVarTruthTableCondition_9 = false;
aVarTruthTableCondition_10 = false;


% Appmode is Standalone or Shift position CAN status is never recived

aVarTruthTableCondition_1 = logical(((Vehicle_status == NETWORK_STANDALONE ) || ( Shift_Position_Can_Status == eSIGNAL_NEVER_RECEIVED)));

% Shift position CAN status is Missing

aVarTruthTableCondition_2 = logical((Shift_Position_Can_Status == eSIGNAL_MISSING));

% Shift position CAN value is 1

aVarTruthTableCondition_3 = logical((Shift_Position_Can_Value == VALUE_ONE));

% Shift position CAN value is 2

aVarTruthTableCondition_4 = logical((Shift_Position_Can_Value == VALUE_TWO));

% Shift position CAN value is 3

aVarTruthTableCondition_5 = logical((Shift_Position_Can_Value == VALUE_THREE));

% Shift position CAN value is 4

aVarTruthTableCondition_6 = logical((Shift_Position_Can_Value == VALUE_FOUR));

% Shift position CAN value is 5

aVarTruthTableCondition_7 = logical((Shift_Position_Can_Value == VALUE_FIVE));

% Shift position CAN value is 6

aVarTruthTableCondition_8 = logical((Shift_Position_Can_Value == VALUE_SIX));

% Shift position CAN value is 7

aVarTruthTableCondition_9 = logical((Shift_Position_Can_Value == VALUE_SEVEN));

% Shift position CAN value is 8

aVarTruthTableCondition_10 = logical((Shift_Position_Can_Value == VALUE_EIGHT));

if (aVarTruthTableCondition_1)
    aFcnTruthTableAction_2();
elseif (aVarTruthTableCondition_2)
    aFcnTruthTableAction_1();
elseif (aVarTruthTableCondition_3)
    aFcnTruthTableAction_3();
elseif (aVarTruthTableCondition_4)
    aFcnTruthTableAction_4();
elseif (aVarTruthTableCondition_5)
    aFcnTruthTableAction_5();
elseif (aVarTruthTableCondition_6)
    aFcnTruthTableAction_6();
elseif (aVarTruthTableCondition_7)
    aFcnTruthTableAction_7();
elseif (aVarTruthTableCondition_8)
    aFcnTruthTableAction_8();
elseif (aVarTruthTableCondition_9)
    aFcnTruthTableAction_9();
elseif (aVarTruthTableCondition_10)
    aFcnTruthTableAction_10();
else % Default
    aFcnTruthTableAction_1();
end

function aFcnTruthTableAction_1()

% Shift position Off

Shift_Position = STATUS_OFF;

function aFcnTruthTableAction_2()

% Maintain Previous Shift position value

Shift_Position = Prev_Shift_Position;

function aFcnTruthTableAction_3()

% Shift position P

Shift_Position = Shift_Pos_RANGE_P;

function aFcnTruthTableAction_4()

% Shift position R

Shift_Position = Shift_Pos_RANGE_R;

function aFcnTruthTableAction_5()

% Shift position N

Shift_Position = Shift_Pos_RANGE_N;

function aFcnTruthTableAction_6()

% Shift position D

Shift_Position = Shift_Pos_RANGE_D;

function aFcnTruthTableAction_7()

% Shift position B

Shift_Position = Shift_Pos_RANGE_B;

function aFcnTruthTableAction_8()

% Shift position M

Shift_Position = Shift_Pos_RANGE_M;

function aFcnTruthTableAction_9()

% Shift position S

Shift_Position = Shift_Pos_RANGE_S;

function aFcnTruthTableAction_10()

% Shift position SD

Shift_Position = Shift_Pos_RANGE_SD;

== matlab function Mdl_Gear/Mdl_Gear_Task_sys/Subsystem/Subsystem1/Subsystem/Gear Step Determination ==
  data: Vehicle_status input; Gear_Step output uint8; STATUS_OFF parameter; Gear_Step_Can_Value input; Gear_Step_Can_Status input; NETWORK_NORMAL parameter; NETWORK_STANDALONE parameter; eSIGNAL_NEVER_RECEIVED parameter; eSIGNAL_MISSING parameter; Prev_Gear_Step input uint8; VALUE_ONE parameter; VALUE_FIFTEEN parameter; VALUE_TEN parameter; VALUE_ZERO parameter
function Gear_Step = fcn(Vehicle_status, STATUS_OFF, Gear_Step_Can_Value, Gear_Step_Can_Status, NETWORK_NORMAL, NETWORK_STANDALONE, eSIGNAL_NEVER_RECEIVED, eSIGNAL_MISSING, Prev_Gear_Step, VALUE_ONE, VALUE_FIFTEEN, VALUE_TEN, VALUE_ZERO)

aVarTruthTableCondition_1 = false;
aVarTruthTableCondition_2 = false;
aVarTruthTableCondition_3 = false;


% Appmode is Standalone or Gear step CAN status is never recived

aVarTruthTableCondition_1 = logical(((Vehicle_status == NETWORK_STANDALONE ) || ( Gear_Step_Can_Status == eSIGNAL_NEVER_RECEIVED)));

% Gear step CAN status is Missing

aVarTruthTableCondition_2 = logical((Gear_Step_Can_Status == eSIGNAL_MISSING));

% Normal Gear Step CAN value is 0 to 15

aVarTruthTableCondition_3 = logical(((Gear_Step_Can_Value >= VALUE_ONE) && (Gear_Step_Can_Value <= VALUE_FIFTEEN)));

if (aVarTruthTableCondition_1)
    aFcnTruthTableAction_2();
elseif (aVarTruthTableCondition_2)
    aFcnTruthTableAction_1();
elseif (aVarTruthTableCondition_3)
    aFcnTruthTableAction_3();
else % Default
    aFcnTruthTableAction_1();
end

function aFcnTruthTableAction_1()

% Gear step is Off

Gear_Step = STATUS_OFF;

function aFcnTruthTableAction_2()

% Maintains Previous Gear step

Gear_Step = Prev_Gear_Step;

function aFcnTruthTableAction_3()

% Gear step is Current Gear Step CAN value

Gear_Step = Gear_Step_Can_Value;
